simulink model "fukt_test"  (R2023b)
settings: Solver=FixedStepAuto  StartTime=0.0  StopTime=inf  FixedStep=0.5  MaxStep=1  MinStep=1  RelTol=1e-3
undefined symbols (not defined in the file or in its folder): BOOL, DINT, OTL, slplc
libraries: arduinolib x3
(part 1 of 6)
settings Model: Creator=pontus  LastModifiedBy=pontus
settings SolverCC: InitialStep=1

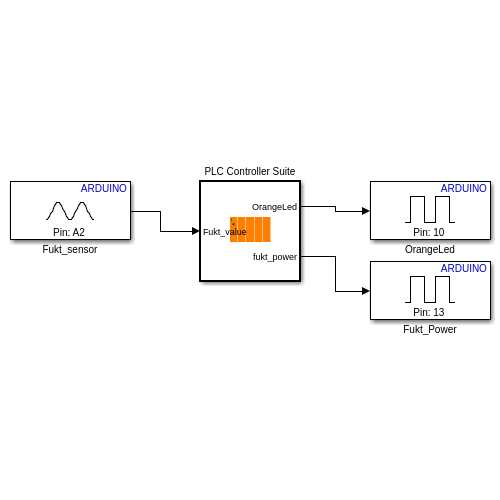
[thumbnail: Simulink's stored preview of the top-level diagram]
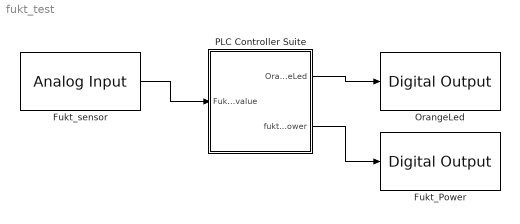
== system fukt_test ==
  Fukt_Power : arduinolib/Digital Output  pinNumber=13  Direction=output  blockPlatform=arduino
  Fukt_sensor : arduinolib/Analog Input  pinNumber=2  ReadResultsOnly=off  ConversionTriggerSource=Software  ExternalTriggerType=uint32( 0 )  OutputDataType=uint16  EnableConversionCompleteNotify=off  EnableOuputStatus=off  SampleTime=-1  blockPlatform=arduino
  OrangeLed : arduinolib/Digital Output  pinNumber=10  Direction=output  blockPlatform=arduino
  PLC Controller Suite : Subsystem  TreatAsAtomicUnit=on  mask{PLCBlockType=PLCController, PLCPOUType=PLC Controller}
      mask init:
      | slplc.callbacks.initController(gcb);
      settings: OpenFcn=slplc.callbacks.openPOUBlock(gcb);
      mask Help: web([docroot '/plccoder/ref/plccontrollersuite' '.html']);
      mask DialogControl PLCBlockTitle Prompt: PLC Controller Block
  wires:
  Fukt_sensor/1 -> PLC Controller Suite/1(Fukt_value)
  PLC Controller Suite/1(OrangeLed) -> OrangeLed/1
  PLC Controller Suite/2(fukt_power) -> Fukt_Power/1

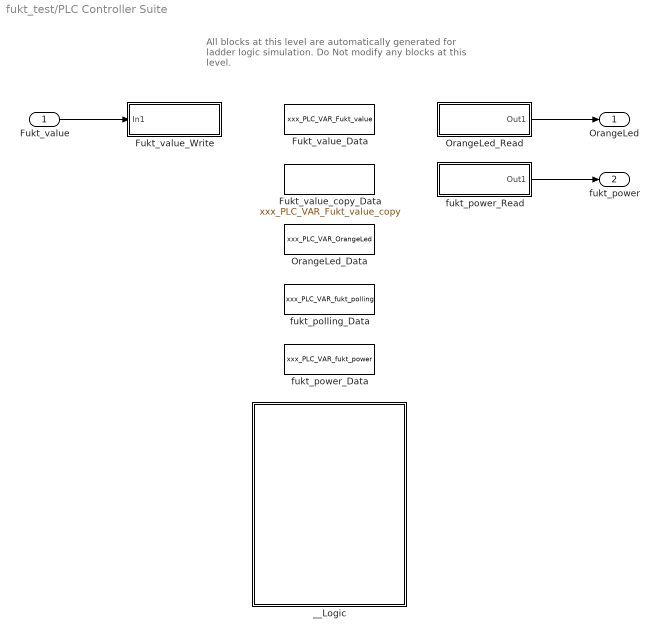
== system fukt_test/PLC Controller Suite ==
  note: All blocks at this level are automatically generated for ladder logic simulation.
      | Do Not modify any blocks at this level.
  Fukt_value : Inport  OutDataTypeStr=uint16  SampleTime=1
  Fukt_value_Data : DataStoreMemory  Tag=POUVariable  Priority=10  DataStoreName=xxx_PLC_VAR_Fukt_value  ShowAdditionalParam=off  OutDataTypeStr=uint16  Dimensions=1
  Fukt_value_Write : Subsystem  Priority=11  DisableCoverage=on  TreatAsAtomicUnit=on  mask{PLCOperandTag=Fukt_value, PLCOperandExpression=xxx_PLC_VAR_Fukt_value, PLCBlockType=VarWrite, PLCPOUType=VarWrite}
      mask prompts: PLCOperandTag "Operand Tag:"
      mask init:
      | slplc.callbacks.initInstruction(gcb);
      mask Help: web([docroot '/plccoder/ref/varwrite' '.html']);
      mask DialogControl PLCBlockTitle Prompt: Variable Write
      mask Display: disp(get_param(gcb, 'PLCOperandTag'));
  Fukt_value_copy_Data : DataStoreMemory  Tag=POUVariable  Priority=10  DataStoreName=xxx_PLC_VAR_Fukt_value_copy  ShowAdditionalParam=off  OutDataTypeStr=uint16  Dimensions=1
  OrangeLed_Data : DataStoreMemory  Tag=POUVariable  Priority=10  DataStoreName=xxx_PLC_VAR_OrangeLed  ShowAdditionalParam=off  OutDataTypeStr=boolean  Dimensions=1
  OrangeLed_Read : Subsystem  Priority=13  DisableCoverage=on  TreatAsAtomicUnit=on  mask{PLCOperandTag=OrangeLed, PLCOperandExpression=xxx_PLC_VAR_OrangeLed, PLCBlockType=VarRead, PLCPOUType=VarRead}
      mask prompts: PLCOperandTag "Operand Tag"
      mask init:
      | block = gcb;
      | maskObj = Simulink.Mask.get(block);
      | maskObj.Display = sprintf('disp(''%s'');', PLCOperandTag);
      | slplc.callbacks.initInstruction(gcb);
      mask Help: web([docroot '/plccoder/ref/varread' '.html']);
      mask DialogControl PLCBlockTitle Prompt: Variable Read
      mask Display: disp('OrangeLed');
  __Logic : Subsystem  Priority=12  TreatAsAtomicUnit=on
  fukt_polling_Data : DataStoreMemory  Tag=POUVariable  Priority=10  DataStoreName=xxx_PLC_VAR_fukt_polling  ShowAdditionalParam=off  OutDataTypeStr=boolean  Dimensions=1
  fukt_power_Data : DataStoreMemory  Tag=POUVariable  Priority=10  DataStoreName=xxx_PLC_VAR_fukt_power  ShowAdditionalParam=off  OutDataTypeStr=boolean  Dimensions=1
  fukt_power_Read : Subsystem  Priority=13  DisableCoverage=on  TreatAsAtomicUnit=on  mask{PLCOperandTag=fukt_power, PLCOperandExpression=xxx_PLC_VAR_fukt_power, PLCBlockType=VarRead, PLCPOUType=VarRead}
      mask prompts: PLCOperandTag "Operand Tag"
      mask init:
      | block = gcb;
      | maskObj = Simulink.Mask.get(block);
      | maskObj.Display = sprintf('disp(''%s'');', PLCOperandTag);
      | slplc.callbacks.initInstruction(gcb);
      mask Help: web([docroot '/plccoder/ref/varread' '.html']);
      mask DialogControl PLCBlockTitle Prompt: Variable Read
      mask Display: disp('fukt_power');
  OrangeLed : Outport  SampleTime=1
  fukt_power : Outport  Port=2  SampleTime=1
  wires:
  Fukt_value/1 -> Fukt_value_Write/1(In1)
  OrangeLed_Read/1(Out1) -> OrangeLed/1
  fukt_power_Read/1(Out1) -> fukt_power/1

== system fukt_test/PLC Controller Suite/Fukt_value_Write ==
  In1 : Inport
  __CoreVarWrite : Subsystem  Tag=CoreVarWriteBlock  DisableCoverage=on  TreatAsAtomicUnit=on  mask{PLCBlockType=CoreVarWrite}
      mask init:
      | slplc.callbacks.initCoreVariable(gcb, 'write');
      mask DialogControl PLCBlockTitle Prompt: Core Variable Write
  wires:
  In1/1 -> __CoreVarWrite/1(u)

== system fukt_test/PLC Controller Suite/OrangeLed_Read ==
  __CoreVarRead : Subsystem  Tag=CoreVarReadBlock  DisableCoverage=on  TreatAsAtomicUnit=on  mask{PLCBlockType=CoreVarRead}
      mask init:
      | slplc.callbacks.initCoreVariable(gcb, 'read');
      mask DialogControl PLCBlockTitle Prompt: Core Variable Read
  Out1 : Outport  VectorParamsAs1DForOutWhenUnconnected=off
  wires:
  __CoreVarRead/1(y) -> Out1/1

== system fukt_test/PLC Controller Suite/__Logic ==
  Controller Tags : Subsystem  Tag=ControllerVariableSS  DisableCoverage=on  TreatAsAtomicUnit=on  mask{PLCVarFukt_valueName=Fukt_value, PLCVarFukt_valueAddress=<empty>, PLCVarFukt_valueMapping=Input Symbol, PLCVarFukt_valuePortIndex=1, PLCVarFukt_valueDataType=uint16, PLCVarFukt_valueSize=1, PLCVarFukt_valueInitialValue=0, PLCVarFukt_valueToDelete=off, PLCVarOrangeLedName=OrangeLed, PLCVarOrangeLedAddress=<empty>, PLCVarOrangeLedMapping=Output Symbol, PLCVarOrangeLedPortIndex=1, PLCVarOrangeLedDataType=boolean, PLCVarOrangeLedSize=1, PLCVarOrangeLedInitialValue=0, PLCVarOrangeLedToDelete=off, PLCVarfukt_powerName=fukt_power, PLCVarfukt_powerAddress=<empty>, PLCVarfukt_powerMapping=Output Symbol, PLCVarfukt_powerPortIndex=2, PLCVarfukt_powerDataType=boolean, PLCVarfukt_powerSize=1, PLCVarfukt_powerInitialValue=0, PLCVarfukt_powerToDelete=off, PLCVarFukt_value_copyName=Fukt_value_copy, PLCVarFukt_value_copyAddress=<empty>, PLCVarFukt_value_copyMapping=Global Variable, PLCVarFukt_value_copyPortIndex=5, PLCVarFukt_value_copyDataType=uint16, PLCVarFukt_value_copySize=1, PLCVarFukt_value_copyInitialValue=0, PLCVarFukt_value_copyToDelete=off, PLCVarfukt_pollingName=fukt_polling, PLCVarfukt_pollingAddress=<empty>, PLCVarfukt_pollingMapping=Global Variable, PLCVarfukt_pollingPortIndex=5, PLCVarfukt_pollingDataType=boolean, PLCVarfukt_pollingSize=1, PLCVarfukt_pollingInitialValue=0, PLCVarfukt_pollingToDelete=off}
      mask init:
      | slplc.callbacks.initControllerVarSS(gcb);
      settings: OpenFcn=slplc.callbacks.openControllerVariableSS(gcb);
      mask Help: web([docroot '/plccoder/ref/controllertags' '.html']);
      mask TypeOptions PLCVarFukt_valueMapping: Global Variable | Input Symbol | Output Symbol
      mask Callback PLCVarFukt_valueMapping: slplc.callbacks.updateControllerVarSS(gcb);
      mask TypeOptions PLCVarFukt_valuePortIndex: 1 | 2 | 3 | 4 | 5
      mask TypeOptions PLCVarOrangeLedMapping: Global Variable | Input Symbol | Output Symbol
      mask Callback PLCVarOrangeLedMapping: slplc.callbacks.updateControllerVarSS(gcb);
      mask TypeOptions PLCVarOrangeLedPortIndex: 1 | 2 | 3 | 4 | 5
      mask TypeOptions PLCVarfukt_powerMapping: Global Variable | Input Symbol | Output Symbol
      mask Callback PLCVarfukt_powerMapping: slplc.callbacks.updateControllerVarSS(gcb);
      mask TypeOptions PLCVarfukt_powerPortIndex: 1 | 2 | 3 | 4 | 5
      mask TypeOptions PLCVarFukt_value_copyMapping: Global Variable | Input Symbol | Output Symbol
      mask Callback PLCVarFukt_value_copyMapping: slplc.callbacks.updateControllerVarSS(gcb);
      mask TypeOptions PLCVarFukt_value_copyPortIndex: 1 | 2 | 3 | 4 | 5
      mask TypeOptions PLCVarfukt_pollingMapping: Global Variable | Input Symbol | Output Symbol
      mask Callback PLCVarfukt_pollingMapping: slplc.callbacks.updateControllerVarSS(gcb);
      mask TypeOptions PLCVarfukt_pollingPortIndex: 1 | 2 | 3 | 4 | 5
      mask DialogControl PLCBlockTitle Prompt: Global Variable and Symbol Spreadsheet
      mask DialogControl PLCVarListHeaderName Prompt: Name
      mask DialogControl PLCVarListHeaderAddress Prompt: Address (At)
      mask DialogControl PLCVarListHeaderMapping Prompt: Mapping Type
      mask DialogControl PLCVarListHeaderPortIndex Prompt: Port
      mask DialogControl PLCVarListHeaderDataType Prompt: Data Type
      mask DialogControl PLCVarListHeaderSize Prompt: Size
      mask DialogControl PLCVarListHeaderInitialValue Prompt: Initial Value
      mask DialogControl PLCVarListHeaderToDelete Prompt: Delete
  Fukt logic : Subsystem  TreatAsAtomicUnit=on  mask{PLCBlockType=Task, PLCPOUType=Task, PLCTaskWatchDog=0}
      mask init:
      | slplc.callbacks.initTask(gcb);
      settings: OpenFcn=slplc.callbacks.openTaskBlock(gcb);
      mask Help: web([docroot '/plccoder/ref/task' '.html']);
      mask DialogControl PLCBlockTitle Prompt: Task
  Fukt sampling : Subsystem  TreatAsAtomicUnit=on  mask{PLCBlockType=Task, PLCPOUType=Task, PLCTaskWatchDog=0}
      mask init:
      | slplc.callbacks.initTask(gcb);
      settings: OpenFcn=slplc.callbacks.openTaskBlock(gcb);
      mask Help: web([docroot '/plccoder/ref/task' '.html']);
      mask DialogControl PLCBlockTitle Prompt: Task
  Up to Parent POU : Subsystem  DisableCoverage=on  TreatAsAtomicUnit=on  mask{PLCBlockType=OpenParentPOU}
      settings: OpenFcn=slplc.callbacks.openParentPOUBlock(gcb);
      mask Help: web([docroot '/plccoder/ref/uptoparentpou' '.html']);
      mask DialogControl PLCBlockTitle Prompt: Add Single Rung

== system fukt_test/PLC Controller Suite/fukt_power_Read ==
  __CoreVarRead : Subsystem  Tag=CoreVarReadBlock  DisableCoverage=on  TreatAsAtomicUnit=on  mask{PLCBlockType=CoreVarRead}
      mask init:
      | slplc.callbacks.initCoreVariable(gcb, 'read');
      mask DialogControl PLCBlockTitle Prompt: Core Variable Read
  Out1 : Outport  VectorParamsAs1DForOutWhenUnconnected=off
  wires:
  __CoreVarRead/1(y) -> Out1/1

== system fukt_test/PLC Controller Suite/Fukt_value_Write/__CoreVarWrite ==
  u : Inport
  DataWrite : DataStoreWrite  DataStoreName=xxx_PLC_VAR_Fukt_value  IndexOptions=Index vector (dialog)  Indices=1  OutputSizes=1
  wires:
  u/1 -> DataWrite/1

== system fukt_test/PLC Controller Suite/OrangeLed_Read/__CoreVarRead ==
  DataRead : DataStoreRead  DataStoreName=xxx_PLC_VAR_OrangeLed  IndexOptions=Index vector (dialog)  Indices=1  OutputSizes=1
  y : Outport  VectorParamsAs1DForOutWhenUnconnected=off
  wires:
  DataRead/1 -> y/1

== system fukt_test/PLC Controller Suite/__Logic/Controller Tags ==

== system fukt_test/PLC Controller Suite/__Logic/Fukt logic ==
  Program : Subsystem  TreatAsAtomicUnit=on  mask{PLCPOUType=Program, PLCPOULanguage=LD, PLCBlockType=LDProgram}
      mask prompts: PLCPOUType "POU Type:"
      mask init:
      | slplc.callbacks.initProgram(gcb);
      settings: OpenFcn=slplc.callbacks.openPOUBlock(gcb);
      mask Help: web([docroot '/plccoder/ref/program' '.html']);
      mask DialogControl PLCBlockTitle Prompt: Program
      mask DialogControl PLCEditPOU Prompt: Edit POU
      mask DialogControl PLCEditInterface Prompt: Edit Variables
  Up to Parent POU : Subsystem  DisableCoverage=on  TreatAsAtomicUnit=on  mask{PLCBlockType=OpenParentPOU}
      settings: OpenFcn=slplc.callbacks.openParentPOUBlock(gcb);
      mask Help: web([docroot '/plccoder/ref/uptoparentpou' '.html']);
      mask DialogControl PLCBlockTitle Prompt: Add Single Rung

== system fukt_test/PLC Controller Suite/__Logic/Fukt sampling ==
  Fuktmätare sampling : Subsystem  TreatAsAtomicUnit=on  mask{PLCPOUType=Program, PLCPOULanguage=LD, PLCBlockType=LDProgram}
      mask prompts: PLCPOUType "POU Type:"
      mask init:
      | slplc.callbacks.initProgram(gcb);
      settings: OpenFcn=slplc.callbacks.openPOUBlock(gcb);
      mask Help: web([docroot '/plccoder/ref/program' '.html']);
      mask DialogControl PLCBlockTitle Prompt: Program
      mask DialogControl PLCEditPOU Prompt: Edit POU
      mask DialogControl PLCEditInterface Prompt: Edit Variables
  Up to Parent POU : Subsystem  DisableCoverage=on  TreatAsAtomicUnit=on  mask{PLCBlockType=OpenParentPOU}
      settings: OpenFcn=slplc.callbacks.openParentPOUBlock(gcb);
      mask Help: web([docroot '/plccoder/ref/uptoparentpou' '.html']);
      mask DialogControl PLCBlockTitle Prompt: Add Single Rung

== system fukt_test/PLC Controller Suite/__Logic/Up to Parent POU ==

== system fukt_test/PLC Controller Suite/fukt_power_Read/__CoreVarRead ==
  DataRead : DataStoreRead  DataStoreName=xxx_PLC_VAR_fukt_power  IndexOptions=Index vector (dialog)  Indices=1  OutputSizes=1
  y : Outport  VectorParamsAs1DForOutWhenUnconnected=off
  wires:
  DataRead/1 -> y/1

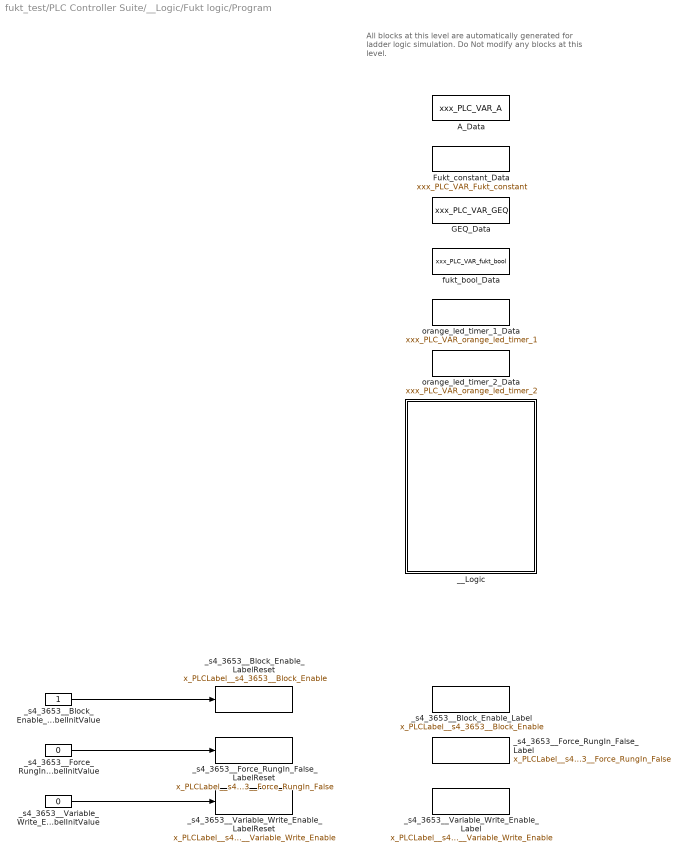
== system fukt_test/PLC Controller Suite/__Logic/Fukt logic/Program ==
  note: All blocks at this level are automatically generated for ladder logic simulation.
      | Do Not modify any blocks at this level.
  A_Data : DataStoreMemory  Tag=POUVariable  Priority=10  DataStoreName=xxx_PLC_VAR_A  InitialValue=1  ShowAdditionalParam=off  OutDataTypeStr=boolean  Dimensions=1
  Fukt_constant_Data : DataStoreMemory  Tag=POUVariable  Priority=10  DataStoreName=xxx_PLC_VAR_Fukt_constant  ShowAdditionalParam=off  OutDataTypeStr=uint16  Dimensions=1
  GEQ_Data : DataStoreMemory  Tag=POUVariable  Priority=10  DataStoreName=xxx_PLC_VAR_GEQ  InitialValue=false  ShowAdditionalParam=off  OutDataTypeStr=BOOL  Dimensions=1
  __Logic : Subsystem  Priority=12  TreatAsAtomicUnit=on
  _s4_3653__Block_Enable_Label : DataStoreMemory  Priority=10  DataStoreName=x_PLCLabel__s4_3653__Block_Enable  InitialValue=1  ShowAdditionalParam=off  OutDataTypeStr=BOOL  Dimensions=1
  _s4_3653__Block_Enable_LabelInitValue : Constant  OutDataTypeStr=BOOL
  _s4_3653__Block_Enable_LabelReset : DataStoreWrite  Priority=11  DataStoreName=x_PLCLabel__s4_3653__Block_Enable  IndexOptions=Index vector (dialog)  Indices=1  OutputSizes=1
  _s4_3653__Force_RungIn_False_Label : DataStoreMemory  Priority=10  DataStoreName=x_PLCLabel__s4_3653__Force_RungIn_False  ShowAdditionalParam=off  OutDataTypeStr=BOOL  Dimensions=1
  _s4_3653__Force_RungIn_False_LabelInitValue : Constant  Value=0  OutDataTypeStr=BOOL
  _s4_3653__Force_RungIn_False_LabelReset : DataStoreWrite  Priority=11  DataStoreName=x_PLCLabel__s4_3653__Force_RungIn_False  IndexOptions=Index vector (dialog)  Indices=1  OutputSizes=1
  _s4_3653__Variable_Write_Enable_Label : DataStoreMemory  Priority=10  DataStoreName=x_PLCLabel__s4_3653__Variable_Write_Enable  ShowAdditionalParam=off  OutDataTypeStr=BOOL  Dimensions=1
  _s4_3653__Variable_Write_Enable_LabelInitValue : Constant  Value=0  OutDataTypeStr=BOOL
  _s4_3653__Variable_Write_Enable_LabelReset : DataStoreWrite  Priority=11  DataStoreName=x_PLCLabel__s4_3653__Variable_Write_Enable  IndexOptions=Index vector (dialog)  Indices=1  OutputSizes=1
  fukt_bool_Data : DataStoreMemory  Tag=POUVariable  Priority=10  DataStoreName=xxx_PLC_VAR_fukt_bool  InitialValue=false  ShowAdditionalParam=off  OutDataTypeStr=BOOL  Dimensions=1
  orange_led_timer_1_Data : DataStoreMemory  Tag=POUVariable  Priority=10  DataStoreName=xxx_PLC_VAR_orange_led_timer_1  InitialValue=TON_InitialValue  ShowAdditionalParam=off  OutDataTypeStr=Bus: TIMER  Dimensions=1
  orange_led_timer_2_Data : DataStoreMemory  Tag=POUVariable  Priority=10  DataStoreName=xxx_PLC_VAR_orange_led_timer_2  InitialValue=TON_InitialValue  ShowAdditionalParam=off  OutDataTypeStr=Bus: TIMER  Dimensions=1
  wires:
  _s4_3653__Block_Enable_LabelInitValue/1 -> _s4_3653__Block_Enable_LabelReset/1
  _s4_3653__Variable_Write_Enable_LabelInitValue/1 -> _s4_3653__Variable_Write_Enable_LabelReset/1
  _s4_3653__Force_RungIn_False_LabelInitValue/1 -> _s4_3653__Force_RungIn_False_LabelReset/1

== system fukt_test/PLC Controller Suite/__Logic/Fukt logic/Up to Parent POU ==

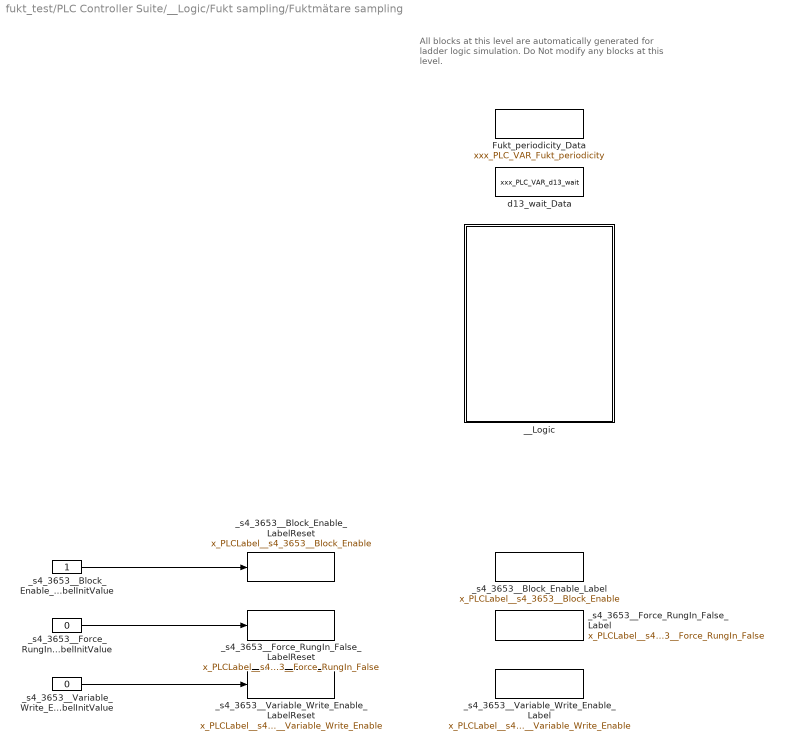
== system fukt_test/PLC Controller Suite/__Logic/Fukt sampling/Fuktmätare sampling ==
  note: All blocks at this level are automatically generated for ladder logic simulation.
      | Do Not modify any blocks at this level.
  Fukt_periodicity_Data : DataStoreMemory  Tag=POUVariable  Priority=10  DataStoreName=xxx_PLC_VAR_Fukt_periodicity  InitialValue=fukt_period  ShowAdditionalParam=off  OutDataTypeStr=Bus: TIMER  Dimensions=1
  __Logic : Subsystem  Priority=12  TreatAsAtomicUnit=on
  _s4_3653__Block_Enable_Label : DataStoreMemory  Priority=10  DataStoreName=x_PLCLabel__s4_3653__Block_Enable  InitialValue=1  ShowAdditionalParam=off  OutDataTypeStr=BOOL  Dimensions=1
  _s4_3653__Block_Enable_LabelInitValue : Constant  OutDataTypeStr=BOOL
  _s4_3653__Block_Enable_LabelReset : DataStoreWrite  Priority=11  DataStoreName=x_PLCLabel__s4_3653__Block_Enable  IndexOptions=Index vector (dialog)  Indices=1  OutputSizes=1
  _s4_3653__Force_RungIn_False_Label : DataStoreMemory  Priority=10  DataStoreName=x_PLCLabel__s4_3653__Force_RungIn_False  ShowAdditionalParam=off  OutDataTypeStr=BOOL  Dimensions=1
  _s4_3653__Force_RungIn_False_LabelInitValue : Constant  Value=0  OutDataTypeStr=BOOL
  _s4_3653__Force_RungIn_False_LabelReset : DataStoreWrite  Priority=11  DataStoreName=x_PLCLabel__s4_3653__Force_RungIn_False  IndexOptions=Index vector (dialog)  Indices=1  OutputSizes=1
  _s4_3653__Variable_Write_Enable_Label : DataStoreMemory  Priority=10  DataStoreName=x_PLCLabel__s4_3653__Variable_Write_Enable  ShowAdditionalParam=off  OutDataTypeStr=BOOL  Dimensions=1
  _s4_3653__Variable_Write_Enable_LabelInitValue : Constant  Value=0  OutDataTypeStr=BOOL
  _s4_3653__Variable_Write_Enable_LabelReset : DataStoreWrite  Priority=11  DataStoreName=x_PLCLabel__s4_3653__Variable_Write_Enable  IndexOptions=Index vector (dialog)  Indices=1  OutputSizes=1
  d13_wait_Data : DataStoreMemory  Tag=POUVariable  Priority=10  DataStoreName=xxx_PLC_VAR_d13_wait  InitialValue=d13_period  ShowAdditionalParam=off  OutDataTypeStr=Bus: TIMER  Dimensions=1
  wires:
  _s4_3653__Block_Enable_LabelInitValue/1 -> _s4_3653__Block_Enable_LabelReset/1
  _s4_3653__Variable_Write_Enable_LabelInitValue/1 -> _s4_3653__Variable_Write_Enable_LabelReset/1
  _s4_3653__Force_RungIn_False_LabelInitValue/1 -> _s4_3653__Force_RungIn_False_LabelReset/1

== system fukt_test/PLC Controller Suite/__Logic/Fukt sampling/Up to Parent POU ==

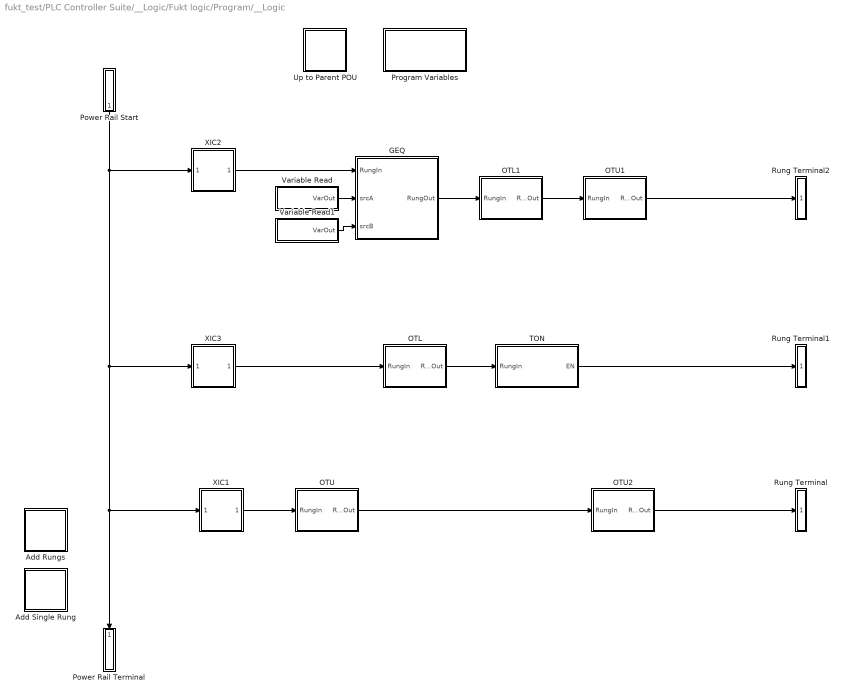
== system fukt_test/PLC Controller Suite/__Logic/Fukt logic/Program/__Logic ==
  Add Rungs : Subsystem  DisableCoverage=on  TreatAsAtomicUnit=on  mask{PLCRungNumberToAdd=2, PLCBlockType=AddRungs}
      mask prompts: PLCRungNumberToAdd "Rung Number:"
      mask Help: web([docroot '/plccoder/ref/addrungs' '.html']);
      mask DialogControl PLCAddRungs Prompt: Add Rungs
      mask DialogControl PLCRungAddButton Prompt: Add
      mask DialogControl PLCRungAddButton Callback: slplc.callbacks.addLadderRungs(gcb);
      mask Display: disp(sprintf(['Add' newline 'Rungs']));
  Add Single Rung : Subsystem  DisableCoverage=on  TreatAsAtomicUnit=on  mask{PLCRungNumberToAdd=1, PLCBlockType=AddSingleRung}
      settings: OpenFcn=slplc.callbacks.addLadderRungs(gcb);
      mask Help: web([docroot '/plccoder/ref/addsinglerung' '.html']);
      mask DialogControl PLCAddRung Prompt: Add Single Rung
      mask Display: disp(sprintf(['Add' newline '1 Rung']));
  GEQ : Subsystem  Priority=5  TreatAsAtomicUnit=on  mask{PLCBlockType=GEQ, PLCPOUType=stdFC}
      mask Help: web([docroot '/plccoder/ref/geq' '.html']);
      mask DialogControl PLCBlockTitle Prompt: Greater Than or Equal To (GEQ)
      mask DialogControl PLCBlockDesc Prompt: Test whether Source A is greater than or equal to Source B.
      mask Display: disp('GEQ');
  OTL : Subsystem  Priority=10  TreatAsAtomicUnit=on  mask{PLCOperandTag=OrangeLed, PLCBlockType=OTL, PLCPOUType=Coil, PLCOperandExpression=xxx_PLC_VAR_OrangeLed}
      mask prompts: PLCOperandTag "Operand Tag:"
      mask init:
      | slplc.callbacks.initInstruction(gcb);
      settings: AttributesFormatString=%<PLCOperandTag>
      mask Help: web([docroot '/plccoder/ref/otl' '.html']);
      mask DialogControl PLCBlockTitle Prompt: Output Latch (OTL)
      mask Display: disp('L');
  OTL1 : Subsystem  Priority=6  TreatAsAtomicUnit=on  mask{PLCOperandTag=fukt_bool, PLCBlockType=OTL, PLCPOUType=Coil, PLCOperandExpression=xxx_PLC_VAR_fukt_bool}
      mask prompts: PLCOperandTag "Operand Tag:"
      mask init:
      | slplc.callbacks.initInstruction(gcb);
      settings: AttributesFormatString=%<PLCOperandTag>
      mask Help: web([docroot '/plccoder/ref/otl' '.html']);
      mask DialogControl PLCBlockTitle Prompt: Output Latch (OTL)
      mask Display: disp('L');
  OTU : Subsystem  Priority=14  TreatAsAtomicUnit=on  mask{PLCOperandTag=OrangeLed, PLCBlockType=OTU, PLCPOUType=Coil, PLCOperandExpression=xxx_PLC_VAR_OrangeLed}
      mask prompts: PLCOperandTag "Operand Tag:"
      mask init:
      | slplc.callbacks.initInstruction(gcb);
      settings: AttributesFormatString=%<PLCOperandTag>
      mask Help: web([docroot '/plccoder/ref/otu' '.html']);
      mask DialogControl PLCBlockTitle Prompt: Output Unlatch (OTU)
      mask Display: disp('U');
  OTU1 : Subsystem  Priority=7  TreatAsAtomicUnit=on  mask{PLCOperandTag=fukt_polling, PLCBlockType=OTU, PLCPOUType=Coil, PLCOperandExpression=xxx_PLC_VAR_fukt_polling}
      mask prompts: PLCOperandTag "Operand Tag:"
      mask init:
      | slplc.callbacks.initInstruction(gcb);
      settings: AttributesFormatString=%<PLCOperandTag>
      mask Help: web([docroot '/plccoder/ref/otu' '.html']);
      mask DialogControl PLCBlockTitle Prompt: Output Unlatch (OTU)
      mask Display: disp('U');
  OTU2 : Subsystem  Priority=15  TreatAsAtomicUnit=on  mask{PLCOperandTag=fukt_bool, PLCBlockType=OTU, PLCPOUType=Coil, PLCOperandExpression=xxx_PLC_VAR_fukt_bool}
      mask prompts: PLCOperandTag "Operand Tag:"
      mask init:
      | slplc.callbacks.initInstruction(gcb);
      settings: AttributesFormatString=%<PLCOperandTag>
      mask Help: web([docroot '/plccoder/ref/otu' '.html']);
      mask DialogControl PLCBlockTitle Prompt: Output Unlatch (OTU)
      mask Display: disp('U');
  Power Rail Start : Subsystem  Priority=1  DisableCoverage=on  TreatAsAtomicUnit=on  mask{PLCBlockType=PowerRailStart}
      mask Help: web([docroot '/plccoder/ref/powerrailstart' '.html']);
      mask DialogControl PLCBlockTitle Prompt: Power Rail Start
      mask DialogControl PLCBlockDesc Prompt: This is the ladder diagram left power rail start block.
  Power Rail Terminal : Subsystem  DisableCoverage=on  TreatAsAtomicUnit=on  mask{PLCBlockType=PowerRailTerminal}
      mask Help: web([docroot '/plccoder/ref/powerrailterminal' '.html']);
      mask DialogControl PLCBlockTitle Prompt: Power Rail Terminal
      mask DialogControl PLCBlockDesc Prompt: This is the ladder diagram left power rail terminal block.
  Program Variables : Subsystem  Tag=ProgramVariableSS  DisableCoverage=on  TreatAsAtomicUnit=on  mask{PLCVarAName=A, PLCVarAScope=Local, PLCVarAPortType=Hidden, PLCVarAPortIndex=9, PLCVarADataType=boolean, PLCVarASize=1, PLCVarAInitialValue=1, PLCVarAToDelete=off, PLCVarFukt_constantName=Fukt_constant, PLCVarFukt_constantScope=Local, PLCVarFukt_constantPortType=Hidden, PLCVarFukt_constantPortIndex=9, PLCVarFukt_constantDataType=uint16, PLCVarFukt_constantSize=1, PLCVarFukt_constantInitialValue=0, PLCVarFukt_constantToDelete=off, PLCVarGEQName=GEQ, PLCVarGEQScope=Local, PLCVarGEQPortType=Hidden, PLCVarGEQPortIndex=9, PLCVarGEQDataType=BOOL, PLCVarGEQSize=1, PLCVarGEQInitialValue=false, PLCVarGEQToDelete=off, PLCVarfukt_boolName=fukt_bool, PLCVarfukt_boolScope=Local, PLCVarfukt_boolPortType=Hidden, PLCVarfukt_boolPortIndex=9, PLCVarfukt_boolDataType=BOOL, PLCVarfukt_boolSize=1, PLCVarfukt_boolInitialValue=false, PLCVarfukt_boolToDelete=off, PLCVarorange_led_timer_1Name=orange_led_timer_1, PLCVarorange_led_timer_1Scope=Local, PLCVarorange_led_timer_1PortType=Hidden, PLCVarorange_led_timer_1PortIndex=9, PLCVarorange_led_timer_1DataType=Bus: TIMER, PLCVarorange_led_timer_1Size=1, PLCVarorange_led_timer_1InitialValue=TON_InitialValue, PLCVarorange_led_timer_1ToDelete=off, PLCVarorange_led_timer_2Name=orange_led_timer_2, PLCVarorange_led_timer_2Scope=Local, PLCVarorange_led_timer_2PortType=Hidden, PLCVarorange_led_timer_2PortIndex=9, PLCVarorange_led_timer_2DataType=Bus: TIMER, PLCVarorange_led_timer_2Size=1, PLCVarorange_led_timer_2InitialValue=TON_InitialValue, PLCVarorange_led_timer_2ToDelete=off, PLCVarFukt_value_copyName=Fukt_value_copy, PLCVarFukt_value_copyScope=External, PLCVarFukt_value_copyPortType=Hidden, PLCVarFukt_value_copyPortIndex=9, PLCVarFukt_value_copyDataType=DINT, PLCVarFukt_value_copySize=-1, PLCVarFukt_value_copyInitialValue=0, PLCVarFukt_value_copyToDelete=off, PLCVarOrangeLedName=OrangeLed, PLCVarOrangeLedScope=External, PLCVarOrangeLedPortType=Hidden, PLCVarOrangeLedPortIndex=9, PLCVarOrangeLedDataType=DINT, PLCVarOrangeLedSize=-1, PLCVarOrangeLedInitialValue=0, PLCVarOrangeLedToDelete=off, PLCVarfukt_pollingName=fukt_polling, PLCVarfukt_pollingScope=External, PLCVarfukt_pollingPortType=Hidden, PLCVarfukt_pollingPortIndex=9, PLCVarfukt_pollingDataType=DINT, PLCVarfukt_pollingSize=-1, PLCVarfukt_pollingInitialValue=0, PLCVarfukt_pollingToDelete=off}
      mask init:
      | slplc.callbacks.initPOUVarSS(gcb);
      settings: OpenFcn=slplc.callbacks.openProgramVariableSS(gcb);
      mask Help: web([docroot '/plccoder/ref/programvariables' '.html']);
      mask TypeOptions PLCVarAScope: Local | External
      mask Callback PLCVarAScope: slplc.callbacks.updatePOUVarSS(gcb);
      mask TypeOptions PLCVarAPortType: Hidden | Inport | Outport
      mask Callback PLCVarAPortType: slplc.callbacks.updatePOUVarSS(gcb);
      mask TypeOptions PLCVarAPortIndex: 1 | 2 | 3 | 4 | 5 | 6 | 7 | 8 | 9
      mask TypeOptions PLCVarFukt_constantScope: Local | External
      mask Callback PLCVarFukt_constantScope: slplc.callbacks.updatePOUVarSS(gcb);
      mask TypeOptions PLCVarFukt_constantPortType: Hidden | Inport | Outport
      mask Callback PLCVarFukt_constantPortType: slplc.callbacks.updatePOUVarSS(gcb);
      mask TypeOptions PLCVarFukt_constantPortIndex: 1 | 2 | 3 | 4 | 5 | 6 | 7 | 8 | 9
      mask TypeOptions PLCVarGEQScope: Local | External
      mask Callback PLCVarGEQScope: slplc.callbacks.updatePOUVarSS(gcb);
      mask TypeOptions PLCVarGEQPortType: Hidden | Inport | Outport
      mask Callback PLCVarGEQPortType: slplc.callbacks.updatePOUVarSS(gcb);
      mask TypeOptions PLCVarGEQPortIndex: 1 | 2 | 3 | 4 | 5 | 6 | 7 | 8 | 9
      mask TypeOptions PLCVarfukt_boolScope: Local | External
      mask Callback PLCVarfukt_boolScope: slplc.callbacks.updatePOUVarSS(gcb);
      mask TypeOptions PLCVarfukt_boolPortType: Hidden | Inport | Outport
      mask Callback PLCVarfukt_boolPortType: slplc.callbacks.updatePOUVarSS(gcb);
      mask TypeOptions PLCVarfukt_boolPortIndex: 1 | 2 | 3 | 4 | 5 | 6 | 7 | 8 | 9
      mask TypeOptions PLCVarorange_led_timer_1Scope: Local | External
      mask Callback PLCVarorange_led_timer_1Scope: slplc.callbacks.updatePOUVarSS(gcb);
      mask TypeOptions PLCVarorange_led_timer_1PortType: Hidden | Inport | Outport
      mask Callback PLCVarorange_led_timer_1PortType: slplc.callbacks.updatePOUVarSS(gcb);
      mask TypeOptions PLCVarorange_led_timer_1PortIndex: 1 | 2 | 3 | 4 | 5 | 6 | 7 | 8 | 9
      mask TypeOptions PLCVarorange_led_timer_2Scope: Local | External
      mask Callback PLCVarorange_led_timer_2Scope: slplc.callbacks.updatePOUVarSS(gcb);
      mask TypeOptions PLCVarorange_led_timer_2PortType: Hidden | Inport | Outport
      mask Callback PLCVarorange_led_timer_2PortType: slplc.callbacks.updatePOUVarSS(gcb);
      mask TypeOptions PLCVarorange_led_timer_2PortIndex: 1 | 2 | 3 | 4 | 5 | 6 | 7 | 8 | 9
      mask TypeOptions PLCVarFukt_value_copyScope: Local | External
      mask Callback PLCVarFukt_value_copyScope: slplc.callbacks.updatePOUVarSS(gcb);
      mask TypeOptions PLCVarFukt_value_copyPortType: Hidden | Inport | Outport
      mask Callback PLCVarFukt_value_copyPortType: slplc.callbacks.updatePOUVarSS(gcb);
      mask TypeOptions PLCVarFukt_value_copyPortIndex: 1 | 2 | 3 | 4 | 5 | 6 | 7 | 8 | 9
      mask TypeOptions PLCVarOrangeLedScope: Local | External
      mask Callback PLCVarOrangeLedScope: slplc.callbacks.updatePOUVarSS(gcb);
      mask TypeOptions PLCVarOrangeLedPortType: Hidden | Inport | Outport
      mask Callback PLCVarOrangeLedPortType: slplc.callbacks.updatePOUVarSS(gcb);
      mask TypeOptions PLCVarOrangeLedPortIndex: 1 | 2 | 3 | 4 | 5 | 6 | 7 | 8 | 9
      mask TypeOptions PLCVarfukt_pollingScope: Local | External
      mask Callback PLCVarfukt_pollingScope: slplc.callbacks.updatePOUVarSS(gcb);
      mask TypeOptions PLCVarfukt_pollingPortType: Hidden | Inport | Outport
      mask Callback PLCVarfukt_pollingPortType: slplc.callbacks.updatePOUVarSS(gcb);
      mask TypeOptions PLCVarfukt_pollingPortIndex: 1 | 2 | 3 | 4 | 5 | 6 | 7 | 8 | 9
      mask DialogControl PLCBlockTitle Prompt: Program Variable Spreadsheet
      mask DialogControl PLCVarListHeaderName Prompt: Name
      mask DialogControl PLCVarListHeaderScope Prompt: Scope
      mask DialogControl PLCVarListHeaderDataType Prompt: Data Type
      mask DialogControl PLCVarListHeaderSize Prompt: Size
      mask DialogControl PLCVarListHeaderInitialValue Prompt: Initial Value
      mask DialogControl PLCVarListHeaderToDelete Prompt: Delete
  Rung Terminal : Subsystem  Priority=16  DisableCoverage=on  TreatAsAtomicUnit=on  mask{PLCRungTerminalIndex=3, PLCBlockType=RungTerminal}
      settings: AttributesFormatString=Rung %<PLCRungTerminalIndex>
      mask Help: web([docroot '/plccoder/ref/rungterminal' '.html']);
      mask DialogControl PLCBlockTitle Prompt: Rung Terminal
      mask DialogControl PLCBlockDescText Prompt: This is the ladder diagram rung terminal.
  Rung Terminal1 : Subsystem  Priority=12  DisableCoverage=on  TreatAsAtomicUnit=on  mask{PLCRungTerminalIndex=2, PLCBlockType=RungTerminal}
      settings: AttributesFormatString=Rung %<PLCRungTerminalIndex>
      mask Help: web([docroot '/plccoder/ref/rungterminal' '.html']);
      mask DialogControl PLCBlockTitle Prompt: Rung Terminal
      mask DialogControl PLCBlockDescText Prompt: This is the ladder diagram rung terminal.
  Rung Terminal2 : Subsystem  Priority=8  DisableCoverage=on  TreatAsAtomicUnit=on  mask{PLCRungTerminalIndex=1, PLCBlockType=RungTerminal}
      settings: AttributesFormatString=Rung %<PLCRungTerminalIndex>
      mask Help: web([docroot '/plccoder/ref/rungterminal' '.html']);
      mask DialogControl PLCBlockTitle Prompt: Rung Terminal
      mask DialogControl PLCBlockDescText Prompt: This is the ladder diagram rung terminal.
  TON : Subsystem  Priority=11  TreatAsAtomicUnit=on  mask{PLCOperandTag=orange_led_timer_1, PLCTimerSampleTime=0.5, PLCBlockType=TON, PLCPOUType=stdFB, PLCOperandAccess=ReadWrite, PLCOperandExpression=xxx_PLC_VAR_orange_led_timer_1}
      mask prompts: PLCOperandTag "Timer Tag:"; PLCTimerSampleTime "Timer Sample Time:"
      mask init:
      | block = gcb;
      | maskObj = Simulink.Mask.get(block);
      | maskObj.Display = sprintf('disp([''%s'' newline newline ''%s'']);', PLCBlockType, PLCOperandTag);
      | slplc.callbacks.initInstruction(block);
      settings: AttributesFormatString=%<PLCBlockType>: %<PLCOperandTag>
      mask Help: web([docroot '/plccoder/ref/ton' '.html']);
      mask DialogControl PLCBlockTitle Prompt: Timer On Delay (TON)
      mask Display: disp(['TON' newline newline 'orange_led_timer_1']);
  Up to Parent POU : Subsystem  DisableCoverage=on  TreatAsAtomicUnit=on  mask{PLCBlockType=OpenParentPOU}
      settings: OpenFcn=slplc.callbacks.openParentPOUBlock(gcb);
      mask Help: web([docroot '/plccoder/ref/uptoparentpou' '.html']);
      mask DialogControl PLCBlockTitle Prompt: Add Single Rung
  Variable Read : Subsystem  Priority=3  TreatAsAtomicUnit=on  mask{PLCOperandTag=Fukt_value_copy, PLCBlockType=VariableRead, PLCOperandAccess=Read, PLCPOUType=VariableRead, PLCOperandExpression=xxx_PLC_VAR_Fukt_value_copy}
      mask prompts: PLCOperandTag "Data Tag:"
      mask init:
      | block = gcb;
      | maskObj = Simulink.Mask.get(block);
      | maskObj.Display = sprintf('disp(''%s'');', PLCOperandTag);
      | slplc.callbacks.initInstruction(block);
      mask Help: web([docroot '/plccoder/ref/variableread' '.html']);
      mask DialogControl PLCBlockTitle Prompt: Data Tag Read
      mask Display: disp('Fukt_value_copy');
  Variable Read1 : Subsystem  Priority=4  TreatAsAtomicUnit=on  mask{PLCOperandTag=Fukt_constant, PLCBlockType=VariableRead, PLCOperandAccess=Read, PLCPOUType=VariableRead, PLCOperandExpression=xxx_PLC_VAR_Fukt_constant}
      mask prompts: PLCOperandTag "Data Tag:"
      mask init:
      | block = gcb;
      | maskObj = Simulink.Mask.get(block);
      | maskObj.Display = sprintf('disp(''%s'');', PLCOperandTag);
      | slplc.callbacks.initInstruction(block);
      mask Help: web([docroot '/plccoder/ref/variableread' '.html']);
      mask DialogControl PLCBlockTitle Prompt: Data Tag Read
      mask Display: disp('Fukt_constant');
  XIC1 : Subsystem  Priority=13  TreatAsAtomicUnit=on  mask{PLCOperandTag=orange_led_timer_1.DN, PLCBlockType=XIC, PLCPOUType=Contact, PLCOperandExpression=xxx_PLC_VAR_orange_led_timer_1.DN}
      mask prompts: PLCOperandTag "Operand Tag:"
      mask init:
      | slplc.callbacks.initInstruction(gcb);
      settings: AttributesFormatString=%<PLCOperandTag>
      mask Help: web([docroot '/plccoder/ref/xic' '.html']);
      mask DialogControl PLCBlockTitle Prompt: Examine If Closed (XIC)
  XIC2 : Subsystem  Priority=2  TreatAsAtomicUnit=on  mask{PLCOperandTag=fukt_polling, PLCBlockType=XIC, PLCPOUType=Contact, PLCOperandExpression=xxx_PLC_VAR_fukt_polling}
      mask prompts: PLCOperandTag "Operand Tag:"
      mask init:
      | slplc.callbacks.initInstruction(gcb);
      settings: AttributesFormatString=%<PLCOperandTag>
      mask Help: web([docroot '/plccoder/ref/xic' '.html']);
      mask DialogControl PLCBlockTitle Prompt: Examine If Closed (XIC)
  XIC3 : Subsystem  Priority=9  TreatAsAtomicUnit=on  mask{PLCOperandTag=fukt_bool, PLCBlockType=XIC, PLCPOUType=Contact, PLCOperandExpression=xxx_PLC_VAR_fukt_bool}
      mask prompts: PLCOperandTag "Operand Tag:"
      mask init:
      | slplc.callbacks.initInstruction(gcb);
      settings: AttributesFormatString=%<PLCOperandTag>
      mask Help: web([docroot '/plccoder/ref/xic' '.html']);
      mask DialogControl PLCBlockTitle Prompt: Examine If Closed (XIC)
  wires:
  OTL/1(RungOut) -> TON/1(RungIn)
  Power Rail Start/1(PowerOut) -> XIC3/1(RungIn), XIC1/1(RungIn), Power Rail Terminal/1(PowerIn), XIC2/1(RungIn)
  OTU/1(RungOut) -> OTU2/1(RungIn)
  XIC3/1(RungOut) -> OTL/1(RungIn)
  XIC1/1(RungOut) -> OTU/1(RungIn)
  XIC2/1(RungOut) -> GEQ/1(RungIn)
  Variable Read/1(VarOut) -> GEQ/2(srcA)
  Variable Read1/1(VarOut) -> GEQ/3(srcB)
  GEQ/1(RungOut) -> OTL1/1(RungIn)
  OTU1/1(RungOut) -> Rung Terminal2/1(RungIn)
  OTL1/1(RungOut) -> OTU1/1(RungIn)
  TON/1(EN) -> Rung Terminal1/1(RungIn)
  OTU2/1(RungOut) -> Rung Terminal/1(RungIn)
